simulink model "Control_Simulation_Lab"  (R2022b)
settings: Solver=VariableStepAuto  StartTime=0.0  StopTime=10.0  RelTol=1e-3
libraries: spsDCVoltageSourceLib x1, spsDCMachineLib x1, spspowerguiLib x1
settings Model: Creator=USER  LastModifiedBy=USER

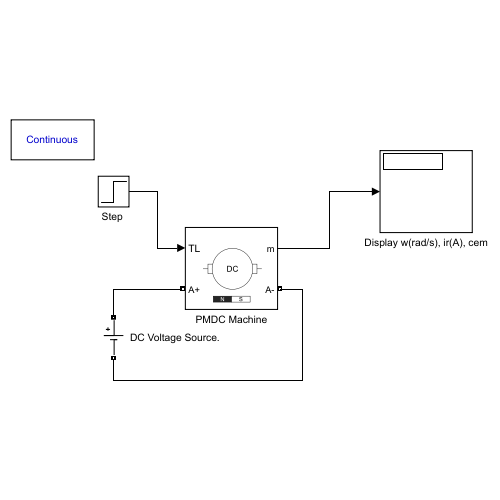
[thumbnail: Simulink's stored preview of the top-level diagram]
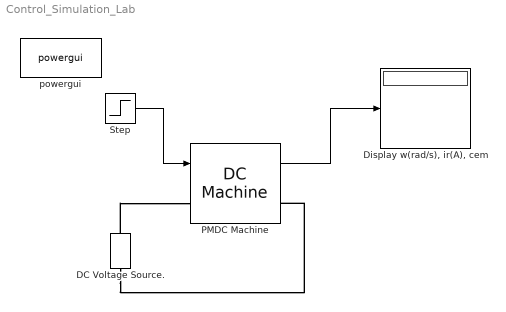
== system Control_Simulation_Lab ==
  DC Voltage Source. : spsDCVoltageSourceLib/DC Voltage Source  Amplitude=24  Measurements=None
  "Display w(rad/s), ir(A), cem" : Display
  PMDC Machine : spsDCMachineLib/DC Machine  PresetModel=No  MechanicalLoad=Torque TL  FieldType=Permanent magnet  ShowDetailedParameters=on  MeasurementBus=off  RLa="[ 0.4  0.001]"  RLf="[ 240  120]"  Laf=1.8  MachineConstant=Torque constant (N.m/A)  Ke=0.3  Kt=0.3  J=0.0009  Bm=0.0025  Tf=0  w0=0  Ifinit=1  TsPowergui=0  TsBlock=-1
  "Step " : Step  SampleTime=0
  powergui : spspowerguiLib/powergui  Priority=1  SimulationMode=Continuous  SampleTime=50e-6  frequency=60  Iterations=50  frequencyindice=0  Pbase=100e6  ErrMax=1e-4  UnitsV=kV  UnitsW=MW  buscounter=0  FunctionMessages=off  echomessages=off  EnableUseOfTLC=off  CurrentSourceSwitches=off  DisableSnubberDevices=off  DisableRonSwitches=off  DisableVfSwitches=off  DisplayEquations=off  AutomaticDiscreteSolvers=off  SolverType=Tustin/Backward Euler (TBE)  Interpol=off  ExternalGateDelay=off  methode=off  Ts=100  x0status=blocks  SPID=on  SwTol=0  HookPort=off  NonlinearTolerance=1e-4  nMaxIteration=100  ContinueOnMaxIteration=off  RestoreLinks=warning  ResistiveCurrentMeasurement=off  Frange=[0:2:500]  Ylog=off  Xlog=on  ShowGrid=off  save=off  variable=ZData  structure=0  ZoomFFT=off  StartTime=0.0  cycles=1  DisplayStyle=1  fundamental=60  FreqAxis=off  MaxFrequency=1000  frequencyindicesteady=1  RmsSteady=1  display=off
  wires:
  "Step "/1 -> PMDC Machine/1
  PMDC Machine/1 -> "Display w(rad/s), ir(A), cem"/1
  connections:
  DC Voltage Source./RConn1 -- PMDC Machine/LConn1
  DC Voltage Source./LConn1 -- PMDC Machine/RConn1
